simulink model "wrapper_2"  (R2024b)
settings: Solver=FixedStepAuto  StartTime=0.0  StopTime=100  FixedStep=T  RelTol=1e-3
settings Model: DataDictionary=wrapper.sldd  Creator=maciej  LastModifiedBy=maciej
settings DebuggingCC: AlgebraicLoopMsg=none

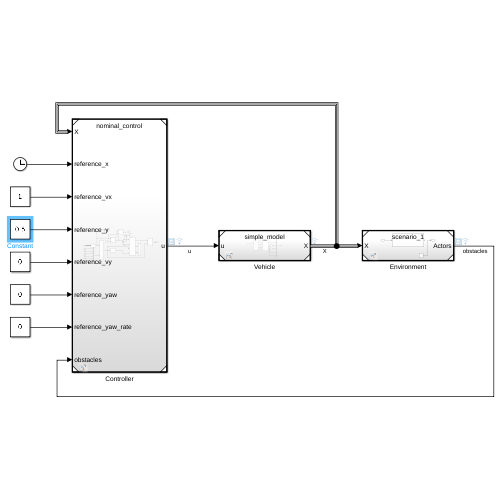
[thumbnail: Simulink's stored preview of the top-level diagram]
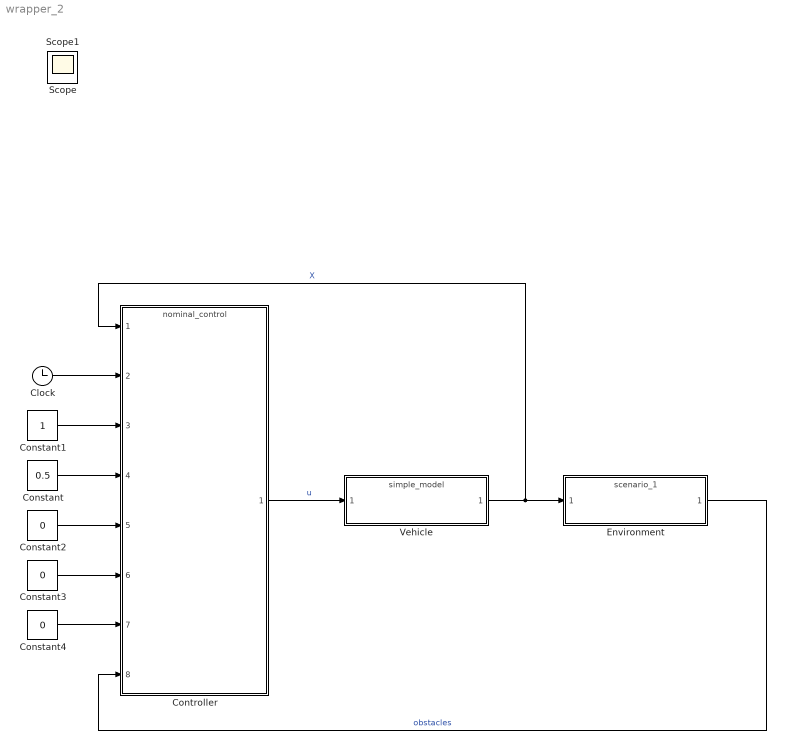
== system wrapper_2 ==
  Clock : Clock
  Constant : Constant  Value=0.5
  Constant1 : Constant
  Constant2 : Constant  Value=0
  Constant3 : Constant  Value=0
  Constant4 : Constant  Value=0
  Controller : ModelReference  ModelNameDialog=nominal_control.slx  SimulationMode=Normal  ModelReferenceVersion=1.193
  Environment : ModelReference  ModelNameDialog=scenario_1.slx  SimulationMode=Normal  ModelReferenceVersion=1.7
  Vehicle : ModelReference  ModelNameDialog=simple_model.slx  SimulationMode=Normal  ModelReferenceVersion=1.27
  Scope : Scope
  Scope1 : Scope
  wires:
  Controller/1 -> Vehicle/1  "u"
  Vehicle/1 -> Environment/1, Controller/1  "X"
  Clock/1 -> Controller/2
  Constant/1 -> Controller/4
  Constant1/1 -> Controller/3
  Constant2/1 -> Controller/5
  Environment/1 -> Controller/8  "obstacles"
  Constant3/1 -> Controller/6
  Constant4/1 -> Controller/7
